simulink model "tryanderror"  (R2025b)
settings: Solver=ode1  StartTime=0.0  StopTime=10.0  RelTol=1e-3
libraries: simulink x10
settings Model: Creator=Odonata-KJ  LastModifiedBy=Odonata-KJ

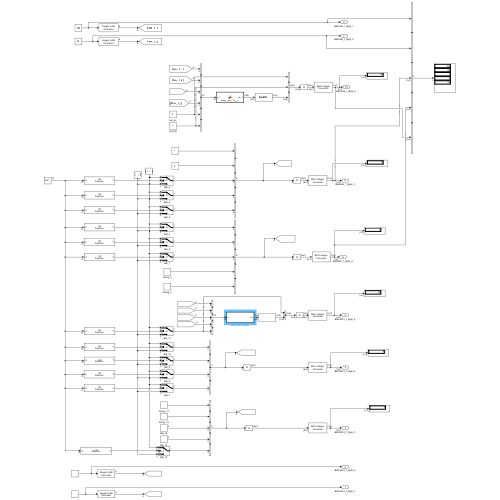
[thumbnail: Simulink's stored preview of the top-level diagram]
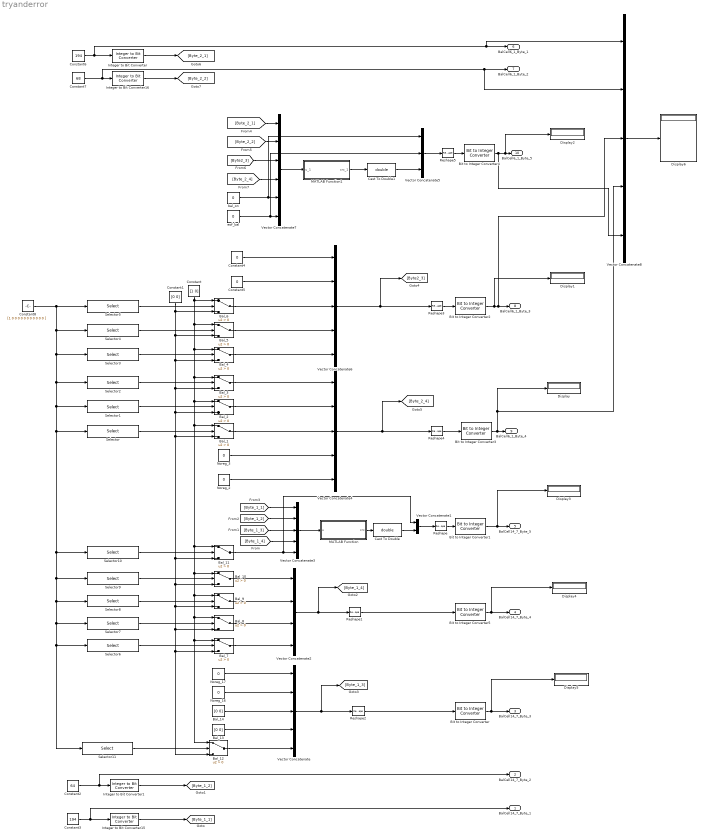
== system tryanderror ==
  Bal_{1..12} (12 alike) : Switch  Criteria=u2 > Threshold  SaturateOnIntegerOverflow=off  InputSameDT=off
  Bal_13 : Constant  Value=[0 0]
  Bal_14 : Constant  Value=[0 0]
  Bit to Integer Converter{,1..5} (6 alike) : simulink/Logic and Bit Operations/Bit to Integer Converter  nbits=8  bitOrder=MSB first  signedOutputValues=Unsigned  outDtype=Inherit via internal rule  outDtypeSigned=Inherit via internal rule
  Cast To Double : DataTypeConversion  OutDataTypeStr=double  SaturateOnIntegerOverflow=off  RndMeth=Floor
  Cast To Double1 : DataTypeConversion  OutDataTypeStr=double  SaturateOnIntegerOverflow=off  RndMeth=Floor
  Constant : Constant  Value=[1 0]
  Constant1 : Constant  Value=[0 0]
  Constant2 : Constant  Value=64
  Constant3 : Constant  Value=194
  Constant4 : Constant  Value=0
  Constant5 : Constant  Value=0
  Constant6 : Constant  Value=194
  Constant7 : Constant  Value=68
  Constant8 : Constant  Value=[1 0 0 0 0 0 0 0 0 0 0 0 ]
  Display{,1..6} (7 alike) : Display
  Integer to Bit Converter{,1,15..16} (4 alike) : simulink/Logic and Bit Operations/Integer to Bit Converter  nbits=8  signedInputValues=Unsigned  bitOrder=MSB first  outDtype=Inherit via internal rule
  MATLAB Function : MATLAB Function  TreatAsAtomicUnit=on
  MATLAB Function1 : MATLAB Function  TreatAsAtomicUnit=on
  Noreg_{2..3,16..17} (4 alike) : Constant  Value=0
  Reshape{,1..5} (6 alike) : Reshape  OutputDimensionality=Customize  OutputDimensions=[8,1]
  Selector : Selector  InputPortWidth=12  IndexOptions=Index vector (dialog)  Indices=1  OutputSizes=1
  Selector1 : Selector  InputPortWidth=12  IndexOptions=Index vector (dialog)  Indices=2  OutputSizes=1
  Selector10 : Selector  InputPortWidth=12  IndexOptions=Index vector (dialog)  Indices=11  OutputSizes=1
  Selector11 : Selector  InputPortWidth=12  IndexOptions=Index vector (dialog)  Indices=12  OutputSizes=1
  Selector2 : Selector  InputPortWidth=12  IndexOptions=Index vector (dialog)  Indices=3  OutputSizes=1
  Selector3 : Selector  InputPortWidth=12  IndexOptions=Index vector (dialog)  Indices=4  OutputSizes=1
  Selector4 : Selector  InputPortWidth=12  IndexOptions=Index vector (dialog)  Indices=5  OutputSizes=1
  Selector5 : Selector  InputPortWidth=12  IndexOptions=Index vector (dialog)  Indices=6  OutputSizes=1
  Selector6 : Selector  InputPortWidth=12  IndexOptions=Index vector (dialog)  Indices=7  OutputSizes=1
  Selector7 : Selector  InputPortWidth=12  IndexOptions=Index vector (dialog)  Indices=8  OutputSizes=1
  Selector8 : Selector  InputPortWidth=12  IndexOptions=Index vector (dialog)  Indices=9  OutputSizes=1
  Selector9 : Selector  InputPortWidth=12  IndexOptions=Index vector (dialog)  Indices=10  OutputSizes=1
  Vector Concatenate{,3..4,6,8} (5 alike) : Concatenate  NumInputs=5
  Vector Concatenate1 : Concatenate
  Vector Concatenate2 : Concatenate  NumInputs=4
  Vector Concatenate5 : Concatenate  NumInputs=3
  Vector Concatenate7 : Concatenate  NumInputs=6
  bal_on : Constant  Value=0
  eof_bal : Constant  Value=0
  BalCell14_7_Byte_1 : Outport
  BalCell14_7_Byte_2 : Outport  Port=2
  BalCell14_7_Byte_3 : Outport  Port=3
  BalCell14_7_Byte_4 : Outport  Port=4
  BalCell14_7_Byte_5 : Outport  Port=5
  BalCell6_1_Byte_1 : Outport  Port=6
  BalCell6_1_Byte_2 : Outport  Port=7
  BalCell6_1_Byte_3 : Outport  Port=8
  BalCell6_1_Byte_4 : Outport  Port=9
  BalCell6_1_Byte_5 : Outport  Port=10
  wires:
  Constant/1 -> Bal_12/1, Bal_7/1, Bal_8/1, Bal_9/1, Bal_10/1, Bal_11/1, Bal_1/1, Bal_2/1, Bal_3/1, Bal_4/1, Bal_5/1, Bal_6/1
  MATLAB Function/1(crc) -> Cast To Double/1
  Vector Concatenate2/1 -> [Byte_1_4], Reshape1/1
  Selector4/1 -> Bal_5/2
  Noreg_16/1 -> Vector Concatenate/2
  Selector7/1 -> Bal_8/2
  Selector2/1 -> Bal_3/2
  Selector5/1 -> Bal_6/2
  Selector3/1 -> Bal_4/2
  Selector6/1 -> Bal_7/2
  Bal_9/1 -> Vector Concatenate2/2
  [Byte_1_4] -> Vector Concatenate3/4
  Bal_14/1 -> Vector Concatenate/3
  Constant3/1 -> BalCell14_7_Byte_1/1, Integer to Bit Converter15/1
  Bal_11/1 -> Vector Concatenate3/5, Vector Concatenate1/1
  Bal_8/1 -> Vector Concatenate2/3
  Bal_10/1 -> Vector Concatenate2/1
  Integer to Bit Converter1/1 -> [Byte_1_2]
  Selector1/1 -> Bal_2/2
  Bit to Integer Converter/1 -> Display5/1, BalCell14_7_Byte_3/1
  Constant1/1 -> Bal_12/3, Bal_7/3, Bal_8/3, Bal_9/3, Bal_10/3, Bal_11/3, Bal_1/3, Bal_2/3, Bal_3/3, Bal_4/3, Bal_5/3, Bal_6/3
  Selector8/1 -> Bal_9/2
  Selector/1 -> Bal_1/2
  Selector9/1 -> Bal_10/2
  Selector11/1 -> Bal_12/2
  [Byte_1_1] -> Vector Concatenate3/1
  Constant8/1 -> Selector11/1, Selector6/1, Selector7/1, Selector8/1, Selector9/1, Selector10/1, Selector/1, Selector1/1, Selector2/1, Selector3/1, Selector4/1, Selector5/1
  Bit to Integer Converter5/1 -> Display4/1, BalCell14_7_Byte_4/1
  Selector10/1 -> Bal_11/2
  Noreg_17/1 -> Vector Concatenate/1
  Constant2/1 -> BalCell14_7_Byte_2/1, Integer to Bit Converter1/1
  Integer to Bit Converter15/1 -> [Byte_1_1]
  Bal_13/1 -> Vector Concatenate/4
  Vector Concatenate/1 -> [Byte_1_3], Reshape2/1
  Bal_7/1 -> Vector Concatenate2/4
  Bal_12/1 -> Vector Concatenate/5
  Constant6/1 -> Vector Concatenate8/1, BalCell6_1_Byte_1/1, Integer to Bit Converter/1
  Vector Concatenate1/1 -> Reshape/1
  Noreg_2/1 -> Vector Concatenate4/5
  Constant7/1 -> Vector Concatenate8/2, BalCell6_1_Byte_2/1, Integer to Bit Converter16/1
  Integer to Bit Converter16/1 -> [Byte_2_2]
  Bal_1/1 -> Vector Concatenate4/3
  Bit to Integer Converter4/1 -> Vector Concatenate8/5, Display2/1, BalCell6_1_Byte_5/1
  Cast To Double1/1 -> Vector Concatenate5/3
  Reshape4/1 -> Bit to Integer Converter3/1
  Constant5/1 -> Vector Concatenate6/2
  Reshape3/1 -> Bit to Integer Converter2/1
  [Byte2_3] -> Vector Concatenate7/3
  [Byte_2_1] -> Vector Concatenate7/1
  Bal_5/1 -> Vector Concatenate6/4
  MATLAB Function1/1(crc_1) -> Cast To Double1/1
  Reshape2/1 -> Bit to Integer Converter/1
  Vector Concatenate4/1 -> [Byte_2_4], Reshape4/1
  Bal_4/1 -> Vector Concatenate6/5
  Integer to Bit Converter/1 -> [Byte_2_1]
  Bit to Integer Converter2/1 -> Display1/1, Vector Concatenate8/3, BalCell6_1_Byte_3/1
  Bal_6/1 -> Vector Concatenate6/3
  Constant4/1 -> Vector Concatenate6/1
  [Byte_2_2] -> Vector Concatenate7/2
  Vector Concatenate7/1 -> MATLAB Function1/1(u_1)
  Cast To Double/1 -> Vector Concatenate1/2
  [Byte_2_4] -> Vector Concatenate7/4
  Vector Concatenate5/1 -> Reshape5/1
  Bit to Integer Converter3/1 -> Vector Concatenate8/4, Display/1, BalCell6_1_Byte_4/1
  [Byte_1_2] -> Vector Concatenate3/2
  Vector Concatenate6/1 -> [Byte2_3], Reshape3/1
  Bal_3/1 -> Vector Concatenate4/1
  Reshape1/1 -> Bit to Integer Converter5/1
  Bit to Integer Converter1/1 -> Display3/1, BalCell14_7_Byte_5/1
  bal_on/1 -> Vector Concatenate7/5, Vector Concatenate5/1
  eof_bal/1 -> Vector Concatenate7/6, Vector Concatenate5/2
  Reshape5/1 -> Bit to Integer Converter4/1
  Bal_2/1 -> Vector Concatenate4/2
  Noreg_3/1 -> Vector Concatenate4/4
  Reshape/1 -> Bit to Integer Converter1/1
  Vector Concatenate3/1 -> MATLAB Function/1(u)
  [Byte_1_3] -> Vector Concatenate3/3
  Vector Concatenate8/1 -> Display6/1

== matlab function tryanderror/MATLAB Function1 ==
  data: u_1 input size=[1 34]; crc_1 output size=[1 6]
function crc_1 = calc_crc6_34_1(u_1)
%#codegen
% Inputs:
%   u   - A 34-element logical or binary array representing the message bits (MSB first).
% Outputs:
%   crc - A 6-element logical array containing the computed 6-bit CRC.

% 1. Define configuration parameters
% Seed: '111000'
seed = logical([1, 1, 1, 0, 0, 0]); 

% Polynomial: x^6 + x^4 + x^3 + 1 -> Binary 1011001. 
% For shift register logic, drop the highest coefficient (x^6):
poly = logical([0, 1, 1, 0, 0, 1]); 

% 2. Initialize internal shift register with seed
reg = seed;

% 3. Process each bit of the 34-bit input frame (Standard Direct Algorithm)
for i = 1:34
    % Determine if a reduction/XOR is needed based on the outgoing bit
    xor_bit = xor(reg(1), u_1(i));
    
    % Shift left by 1 position
    reg = [reg(2:6), false];
    
    % Apply polynomial if the XOR condition is true
    if xor_bit
        reg = xor(reg, poly);
    end
end
crc_1 = reg;

== matlab function tryanderror/MATLAB Function ==
  data: u input size=[1 34]; crc output size=[1 6]
function crc = calc_crc6_34(u)
%#codegen
% Inputs:
%   u   - A 34-element logical or binary array representing the message bits (MSB first).
% Outputs:
%   crc - A 6-element logical array containing the computed 6-bit CRC.

% 1. Define configuration parameters
% Seed: '111000'
seed = logical([1, 1, 1, 0, 0, 0]); 

% Polynomial: x^6 + x^4 + x^3 + 1 -> Binary 1011001. 
% For shift register logic, drop the highest coefficient (x^6):
poly = logical([0, 1, 1, 0, 0, 1]); 

% 2. Initialize internal shift register with seed
reg = seed;

% 3. Process each bit of the 34-bit input frame (Standard Direct Algorithm)
for i = 1:34
    % Determine if a reduction/XOR is needed based on the outgoing bit
    xor_bit = xor(reg(1), u(i));
    
    % Shift left by 1 position
    reg = [reg(2:6), false];
    
    % Apply polynomial if the XOR condition is true
    if xor_bit
        reg = xor(reg, poly);
    end
end
crc=reg;
